simulink model "LHVRT_DipGenTester"  (Simulink 8.1)
settings: Solver=ode45  SolverMode=SingleTasking  StartTime=0.0  StopTime=0.4  RelTol=1e-3
InitFcn:
  | Ts = 50e-6
undefined symbols (not defined in the file or in its folder): D11, Delta
libraries: powerlib x21, powerlib_meascontrol x2, powerlib_extras x1
settings Model: Creator=anony  LastModifiedBy=anony  CovMetricSettings=dwe  CovHtmlReporting=off  covSaveCumulativeToWorkspaceVar=off  CovSaveSingleToWorkspaceVar=off  CovExternalEMLEnable=on
settings DataIOCC: LimitDataPoints=off  SaveFormat=StructureWithTime  SignalLoggingSaveFormat=Dataset  ReturnWorkspaceOutputs=on
settings OptimizationCC: ExpressionDepthLimit=128
settings DebuggingCC: UnderspecifiedInitializationDetection=Simplified  MergeDetectMultiDrivingBlocksExec=error  SolverPrmCheckMsg=none  FcnCallInpInsideContextMsg=EnableAllAsError  FrameProcessingCompatibilityMsg=error  StateNameClashWarn=none  SFUnexpectedBacktrackingDiag=error  SFNoUnconditionalDefaultTransitionDiag=error
settings HardwareCC: ProdBitPerPointer=64  ProdLargestAtomicFloat=Float  ProdIntDivRoundTo=Zero  ProdEndianess=LittleEndian  ProdHWDeviceType=Specified
settings ModelReferenceCC: PropagateSignalLabelsOutOfModel=on
settings SFSimCC: SimUseLocalCustomCode=on
settings RTWCC: RTWUseLocalCustomCode=on
settings GRTTargetCC: CodeReplacementLibrary=C99 (ISO)  CombineOutputUpdateFcns=on  GRTInterface=off

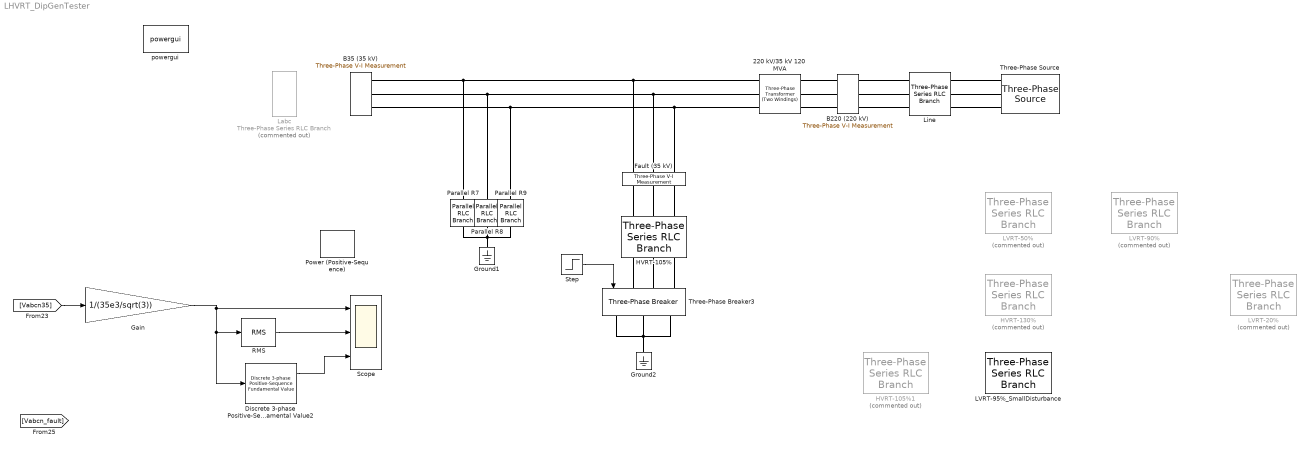
== system LHVRT_DipGenTester ==
  220 kV/35 kV 120 MVA : powerlib/Elements/Three-Phase Transformer (Two Windings)  Winding1Connection=Yg  Winding2Connection=Delta (D11)  CoreType=Three single-phase transformers  SetSaturation=off  Hysteresis=off  DataFile='basic_model'  SetInitialFlux=off  Measurements=None  UNITS=pu  NominalPower=[240e6 50 ]  Winding1="[ 230e3  0.0012   0.07]  %[ 230e3  0.07/30   0.07 ]"  Winding2="[ 35e3  0.0012   0.07]  %[ 38.5e3  0.07/30  0.07]"  Rm=1.7778e3  Lm=250  L0=0.5  Saturation="[ 0,0  ;  0.005,1.2  ;  1.0,1.4 ]"  InitialFluxes=[ 0.8 , -0.8 , 0.7 ]  BreakLoop=off  DiscreteSolver=Trapezoidal iterative  DataType=off  TransfoNumber=0
  B220 (220 kV) : powerlib/Measurements/Three-Phase V-I Measurement  VoltageMeasurement=phase-to-ground  SetLabelV=on  LabelV=Vabcn220  Vpu=off  VpuLL=off  CurrentMeasurement=yes  SetLabelI=on  LabelI=Iabc220  Ipu=off  Pbase=99e6  Vbase=220e3  OutputType=Complex  PhasorSimulation=off  PSBequivalent=0
  B35 (35 kV) : powerlib/Measurements/Three-Phase V-I Measurement  VoltageMeasurement=phase-to-ground  SetLabelV=on  LabelV=Vabcn35  Vpu=off  VpuLL=off  CurrentMeasurement=yes  SetLabelI=on  LabelI=Iabc35  Ipu=off  Pbase=99e6  Vbase=220e3  OutputType=Complex  PhasorSimulation=off  PSBequivalent=0
  Discrete 3-phase Positive-Sequence Fundamental Value2 : powerlib_extras/Discrete Measurements/Discrete 3-phase Positive-Sequence Fundamental Value  Freq=50  Par_Init=[0 0]  Ts=Ts
  Fault (35 kV) : powerlib/Measurements/Three-Phase V-I Measurement  VoltageMeasurement=phase-to-ground  SetLabelV=on  LabelV=Vabcn_fault  Vpu=off  VpuLL=off  CurrentMeasurement=yes  SetLabelI=on  LabelI=Iabc_fault  Ipu=off  Pbase=99e6  Vbase=220e3  OutputType=Complex  PhasorSimulation=off  PSBequivalent=0
  Gain : Gain  Gain=1/(35e3/sqrt(3))
  Ground1 : powerlib/Elements/Ground  LConnTagsString=a
  Ground2 : powerlib/Elements/Ground  LConnTagsString=a
  HVRT-105% : powerlib/Elements/Three-Phase Series RLC Branch  LConnTagsString=A|B|C  RConnTagsString=A|B|C  BranchType=RC  Resistance=1  Inductance=0.077873/300 * 70  Capacitance=1e-4 * 2.1  Measurements=None
  HVRT-105%1 : powerlib/Elements/Three-Phase Series RLC Branch  Commented=on  LConnTagsString=A|B|C  RConnTagsString=A|B|C  BranchType=RC  Resistance=1  Inductance=0.077873/300 * 70  Capacitance=1e-4 * 2.1  Measurements=None
  HVRT-130% : powerlib/Elements/Three-Phase Series RLC Branch  Commented=on  LConnTagsString=A|B|C  RConnTagsString=A|B|C  BranchType=RC  Resistance=1  Inductance=0.077873/300 * 70  Capacitance=10e-4  Measurements=None
  LVRT-20% : powerlib/Elements/Three-Phase Series RLC Branch  Commented=on  LConnTagsString=A|B|C  RConnTagsString=A|B|C  BranchType=RL  Resistance=0.06  Inductance=0.077873/142  Capacitance=0.077873*2.4  Measurements=None
  LVRT-50% : powerlib/Elements/Three-Phase Series RLC Branch  Commented=on  LConnTagsString=A|B|C  RConnTagsString=A|B|C  BranchType=RL  Resistance=0.06  Inductance=0.077873/33.6  Capacitance=0.077873*2.4  Measurements=None
  LVRT-90% : powerlib/Elements/Three-Phase Series RLC Branch  Commented=on  LConnTagsString=A|B|C  RConnTagsString=A|B|C  BranchType=RL  Resistance=0.06  Inductance=0.077873/3.7  Capacitance=0.077873*2.4  Measurements=None
  LVRT-95%_SmallDisturbance : powerlib/Elements/Three-Phase Series RLC Branch  LConnTagsString=A|B|C  RConnTagsString=A|B|C  BranchType=RL  Resistance=0.06  Inductance=0.077873/1.75  Capacitance=0.077873*2.4  Measurements=None
  "Labc " : powerlib/Elements/Three-Phase Series RLC Branch  Commented=on  LConnTagsString=A|B|C  RConnTagsString=A|B|C  BranchType=L  Resistance=0.3  Inductance=46.5e-3  Capacitance=1e-6  Measurements=None
  Line : powerlib/Elements/Three-Phase Series RLC Branch  LConnTagsString=A|B|C  RConnTagsString=A|B|C  BranchType=RL  Resistance=2.1 * 0.03616  Inductance=2.1 * 0.305/(100*pi)  Capacitance=10e-4  Measurements=None
  Parallel R7 : powerlib/Elements/Parallel RLC Branch  LConnTagsString=a  RConnTagsString=__new0  BranchType=R  Resistance=1e9  Inductance=1000  SetiL0=off  InitialCurrent=0  Capacitance=1e-6  Setx0=off  InitialVoltage=0  Measurements=None
  Parallel R8 : powerlib/Elements/Parallel RLC Branch  LConnTagsString=a  RConnTagsString=__new0  BranchType=R  Resistance=1e9  Inductance=1000  SetiL0=off  InitialCurrent=0  Capacitance=1e-6  Setx0=off  InitialVoltage=0  Measurements=None
  Parallel R9 : powerlib/Elements/Parallel RLC Branch  LConnTagsString=a  RConnTagsString=__new0  BranchType=R  Resistance=1e9  Inductance=1000  SetiL0=off  InitialCurrent=0  Capacitance=1e-6  Setx0=off  InitialVoltage=0  Measurements=None
  Power (Positive-Sequence) : powerlib_meascontrol/Measurements/Power (Positive-Sequence)  Freq=50  Vinit=[0, 0]  Iinit=[0, 0]  Ts=0
  RMS : powerlib_meascontrol/Measurements/RMS  TrueRMS=on  Freq=50  RMSInit=0  Ts=0  treatSBRowAsCol=off
  Scope : Scope  NumInputPorts=3
      settings: TimeRange=auto  MaxDataPoints=5000  SaveToWorkspace=off  SaveName=ScopeData  YMin=-2.63877~1.04932~-0.19184  YMax=2.39382~1.05108~1.72657  SampleTime=-1
  Step : Step  Time=0.2  SampleTime=0
  Three-Phase Breaker3 : powerlib/Elements/Three-Phase Breaker  InitialState=open  SwitchA=on  SwitchB=on  SwitchC=on  SwitchTimes=2  External=on  BreakerResistance=0.001  SnubberResistance=1e6  SnubberCapacitance=inf  Measurements=None
  Three-Phase Source : powerlib/Electrical Sources/Three-Phase Source  InternalConnection=Yg  VoltagePhases=off  Voltage=230e3  PhaseAngle=0  Voltage_phases=[25e3 25e3 25e3]/sqrt(3)  PhaseAngles_phases=[0 -120 +120]  Frequency=50  NonIdealSource=on  SpecifyImpedance=off  Resistance=1e-6  Inductance=1e-6  ShortCircuitLevel=5682e6  BaseVoltage=230e3  XRratio=9  BusType=swing  Pref=0  Qref=0  Prefabc=[10e3, 10e3, 10e3]  Qrefabc=[0, 0, 0]  Qmin=-inf  Qmax=inf
  powergui : powerlib/powergui  Priority=1  SimulationMode=Discrete  SampleTime=Ts  frequency=60  Iterations=50  frequencyindice=50  Pbase=100e6  ErrMax=1e-4  UnitsV=kV  UnitsW=MW  buscounter=0  FunctionMessages=off  echomessages=off  EnableUseOfTLC=off  CurrentSourceSwitches=off  DisableSnubberDevices=off  DisableRonSwitches=off  DisableVfSwitches=off  DisplayEquations=off  AutomaticDiscreteSolvers=off  SolverType=Tustin  Interpol=off  ExternalGateDelay=off  methode=off  Ts=0  x0status=blocks  SPID=off  SwTol=0  HookPort=off  NonlinearTolerance=1e-4  nMaxIteration=100  ContinueOnMaxIteration=off  RestoreLinks=warning  ResistiveCurrentMeasurement=off  Frange=[0:2:500]  Ylog=off  Xlog=on  ShowGrid=off  save=off  variable=ZData  structure=0  ZoomFFT=off  StartTime=0.0  cycles=1  DisplayStyle=1  fundamental=60  FreqAxis=off  MaxFrequency=1000  frequencyindicesteady=1  RmsSteady=1  display=off
  wires:
  Step/1 -> Three-Phase Breaker3/1
  RMS/1 -> Scope/2
  [Vabcn35] -> Gain/1
  Gain/1 -> Discrete 3-phase Positive-Sequence Fundamental Value2/1, RMS/1, Scope/1
  Discrete 3-phase Positive-Sequence Fundamental Value2/1 -> Scope/3
  connections:
  Parallel R7/LConn1 -- Fault (35 kV)/LConn1 -- 220 kV/35 kV 120 MVA/RConn1 -- B35 (35 kV)/RConn1
  Parallel R8/LConn1 -- Fault (35 kV)/LConn2 -- 220 kV/35 kV 120 MVA/RConn2 -- B35 (35 kV)/RConn2
  Parallel R9/LConn1 -- Fault (35 kV)/LConn3 -- 220 kV/35 kV 120 MVA/RConn3 -- B35 (35 kV)/RConn3
  Parallel R8/RConn1 -- Parallel R7/RConn1 -- Ground1/LConn1 -- Parallel R9/RConn1
  220 kV/35 kV 120 MVA/LConn2 -- B220 (220 kV)/LConn2
  220 kV/35 kV 120 MVA/LConn3 -- B220 (220 kV)/LConn3
  220 kV/35 kV 120 MVA/LConn1 -- B220 (220 kV)/LConn1
  Three-Phase Breaker3/RConn2 -- Ground2/LConn1 -- Three-Phase Breaker3/RConn3 -- Three-Phase Breaker3/RConn1
  HVRT-105%/RConn3 -- Three-Phase Breaker3/LConn3
  HVRT-105%/RConn1 -- Three-Phase Breaker3/LConn1
  HVRT-105%/RConn2 -- Three-Phase Breaker3/LConn2
  HVRT-105%/LConn1 -- Fault (35 kV)/RConn1
  HVRT-105%/LConn2 -- Fault (35 kV)/RConn2
  HVRT-105%/LConn3 -- Fault (35 kV)/RConn3
  Line/RConn1 -- B220 (220 kV)/RConn1
  Line/RConn2 -- B220 (220 kV)/RConn2
  Line/LConn1 -- Three-Phase Source/RConn1
  Line/LConn2 -- Three-Phase Source/RConn2
  Line/LConn3 -- Three-Phase Source/RConn3
  Line/RConn3 -- B220 (220 kV)/RConn3
